simulink model "HeatingSystem"  (R2017a)
settings: Solver=FixedStepAuto  StartTime=0.0  StopTime=100  FixedStep=0.1  MaxStep=0.1  RelTol=1e-3
PreLoadFcn:
  | load ('parameters\parameters.mat');
libraries: simulink x1
settings Model: Creator=xiaodong  LastModifiedBy=xiaodong
settings DataIOCC: SaveFormat=Array  SaveTime=off

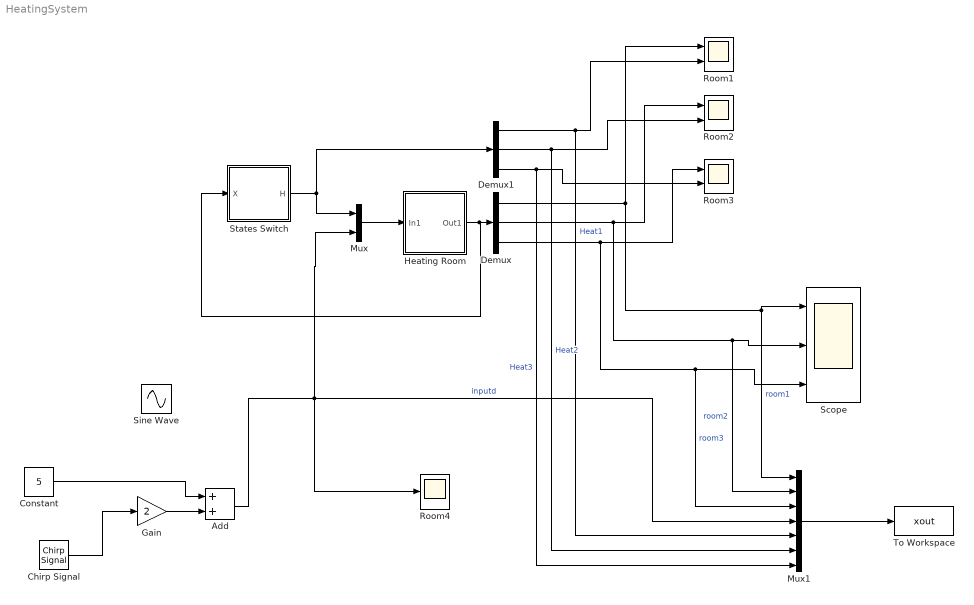
== system HeatingSystem ==
  Add : Sum
  Chirp Signal : simulink/Sources/Chirp Signal  f1=0.001  T=100  f2=0.01
  Constant : Constant  Value=5
  Demux : Demux  Outputs=3
  Demux1 : Demux  Outputs=3
  Gain : Gain  Gain=2
  Heating Room : Subsystem
  Mux : Mux  Inputs=2
  Mux1 : Mux  Inputs=7
  Room1 : Scope  NumInputPorts=2
  Room2 : Scope  NumInputPorts=2
  Room3 : Scope  NumInputPorts=2
  Room4 : Scope
  Scope : Scope  NumInputPorts=3
  Sine Wave : Sin  Amplitude=1.5  Bias=4  Frequency=0.1  SampleTime=0
  States Switch : Stateflow chart  TreatAsAtomicUnit=on
  To Workspace : ToWorkspace  VariableName=xout  SampleTime=0.1
  wires:
  Demux/1 -> Room1/1, Mux1/1, Scope/1  "room1"
  Demux/3 -> Room3/1, Mux1/3, Scope/3  "room3"
  Heating Room/1(Out1) -> States Switch/1(X), Demux/1
  Mux/1 -> Heating Room/1(In1)
  States Switch/1(H) -> Mux/1, Demux1/1
  Demux1/1 -> Mux1/5, Room1/2  "Heat1"
  Demux1/3 -> Mux1/7, Room3/2  "Heat3"
  Demux/2 -> Room2/1, Mux1/2, Scope/2  "room2"
  Demux1/2 -> Mux1/6, Room2/2  "Heat2"
  Add/1 -> Mux1/4, Room4/1, Mux/2  "inputd"
  Mux1/1 -> To Workspace/1
  Constant/1 -> Add/1
  Chirp Signal/1 -> Gain/1
  Gain/1 -> Add/2

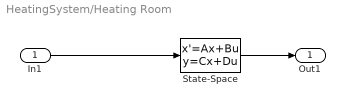
== system HeatingSystem/Heating Room ==
  In1 : Inport
  State-Space : StateSpace  A=|  B="[    0.90000         0           0    0.03000;         0    0.70000       0    0.02000;         0         0   1.10000     0.05000]"  C=eye(3,3)  D=zeros(3,4)  X0=[10 10 10]'
      | [  -0.1000    0.03000    0.04000;
      |     0.03000   -0.10000    0.05000 ;
      |     0.04000    0.05000   -0.14]
  Out1 : Outport
  wires:
  In1/1 -> State-Space/1
  State-Space/1 -> Out1/1

== stateflow chart HeatingSystem/States Switch ==
  settings: updateMethod=DISCRETE  sampleTime=0.1
  state s1
    state s1_2
      entry:
      H(1) = 1;
      H(2) = 0;
      H(3) = 0;
      %out=H;
      %during:
      %out = H;
    state s1_1
      entry:
      H(1) = 0;
      H(2) = 0;
      H(3) = 0;
      %out=H;
      %during:
      %out = H;
    (default) -> s1_2
    s1_1 -> s1_2 : [X(1)<=20]{H(1)=1;}
    s1_2 -> s1_1 : [X(1)>=21]{H(1)=0;}
  state s2
    state s2_2
      entry:
      H(1) = 0;
      H(2) = 1;
      H(3) = 0;
      %out=H;
      %during:
      %out = H;
    state s2_1
      entry:
      H(1) = 0;
      H(2) = 0;
      H(3) = 0;
      %out=H;
      %during:
      %out = H;
    (default) -> s2_2
    s2_1 -> s2_2 : [X(2)<=19]{H(2)=1;}
    s2_2 -> s2_1 : [X(2)>=21]{H(2)=0;}
  state s3
    state s3_1
      entry:
      H(1) = 0;
      H(2) = 0;
      H(3) = 0;
      %out=H;
      %during:
      %out = H;
    state s3_2
      entry:
      H(1) = 0;
      H(2) = 0;
      H(3) = 1;
      %out=H;
      %during:
      %out = H;
    (default) -> s3_2
    s3_1 -> s3_2 : [X(3)<=19]{H(3)=1;}
    s3_2 -> s3_1 : [X(3)>=22]{H(3)=0;}
  (default) -> s2 : {H = [0,0,0]';}
  s1 -> s2 : [X(2)<=get(2)&&(X(1)-X(2)>=dif(2))]
  s3 -> s1 : [X(1)<=get(1)&&(X(3)-X(1)>=dif(1))]
  s2 -> s3 : [X(3)<=get(3)&&(X(2)-X(3)>=dif(3))]
  data: dif constant double size=3 =[2 3 2]'; X input size=3; get constant double size=3 =[16,16,15]'; H output size=3
